simulink model "aIEEE13bus_with_solar_13bus_pl_1day"  (R2025a)
settings: Solver=ode4  StartTime=0.0  StopTime=168  FixedStep=5e-6  MaxStep=1e-4  RelTol=1e-4
InitFcn:
  | a=1; % Loading Factor
  | Ts=50e-6;
  | % phase to sequence conversion of RXB matrices
  | c=1*exp(sqrt(-1)*(120*pi/180));
  | T=[1 1 1;1 c*c c;1 c c*c];
  | Tinv=1/3*[1 1 1;1 c c*c;1 c*c c];
  | 
  | % Simulation data for the IEEE 13 Node Test Feeder model
  | mi2km = 1.60934;%  miles to km conversion
  | ft2km = 0.0003048; % feet to km conversion
  | ms2F = 1*1e-6/(2*pi*60);% microsiemens to Farads conversion
  | 
  | 
  | %% Configuration 601
  | % Series Resitance and Reactance - ohm/mile
  | R_601 = [0.3465 0.1560 0.1580;0.1560 0.3375 0.1535;0.1580 0.1535 0.3414];
  | X_601 = [1.1079 0.5017 0.4236;0.5017 1.0478 0.3849;0.4236 0.3849 1.0348];
  | % charging susceptance - microsiemens/mile
  | B_601 = [6.2998 -1.9958 -1.2595;-1.9958 5.9597 -0.7417;-1.2595 -0.7417 5.6386];
  | 
  | R_601 = R_601/mi2km;
  | Rseq=Tinv*R_601*T;
  | R1_601=Rseq(2,2);R0_601=Rseq(1,1);
  | 
  | L_601 = (X_601/(2*pi*60))/mi2km;
  | Lseq=Tinv*L_601*T;
  | L1_601=Lseq(2,2);L0_601=Lseq(1,1);
  | 
  | C_601 =(B_601*ms2F)/mi2km;
  | Cseq=Tinv*C_601*T;
  | C1_601=Cseq(2,2);C0_601=Cseq(1,1);
  | 
  | %% Configuration 602 - series reactance - ohm/mile
  | R_602 = [0.7526 0.1580 0.1560;0.1580 0.7475 0.1535;0.1560 0.1535 0.7436];
  | X_602 = [1.1814 0.4236 0.5017;0.4236 1.1983 0.3849;0.5017 0.3849 1.2112];
  | % charging susceptance - microsiemens/mile
  | B_602 = [5.6990 -1.0817 -1.6905;-1.0817 5.1795 -0.6588;-1.6905 -0.6588 5.4246];
  | 
  | R_602 = R_602/mi2km;
  | Rseq=Tinv*R_602*T;
  | R1_602=Rseq(2,2);R0_602=Rseq(1,1);
  | 
  | L_602 = (X_602/(2*pi*60))/mi2km;
  | Lseq=Tinv*L_602*T;
  | L1_602=Lseq(2,2);L0_602=Lseq(1,1);
  | 
  | C_602 =(B_602*ms2F)/mi2km;
  | Cseq=Tinv*C_602*T;
  | C1_602=Cseq(2,2);C0_602=Cseq(1,1);
  | %% Configuration 603 - series reactance - ohm/mile
  | R_603 = [0 0 0;0 1.3294 0.2066;0 0.2066 1.3238];
  | X_603 = [0 0 0;0 1.3471 0.4591;0 0.4591 1.3569];
  | % charging susceptance - microsiemens/mile
  | B_603 = [0 0 0;0 4.7097 -0.8999;0 -0.8999 4.6658];
  | 
  | % convert for SPS
  | R_603 = R_603/mi2km;
  | Rseq=Tinv*R_603*T;
  | R1_603=Rseq(2,2);R0_603=Rseq(1,1);
  | 
  | ... (+71 lines)
undefined symbols (not defined in the file or in its folder): D1, Delta, find_system, gcbh, sps_rtmsupport, Ts_Control, Ts_Power
libraries: spsSeriesRLCBranchLib x93, spsGroundLib x57, spsVoltageMeasurementLib x52, spsFourierLib x30, spsThreePhaseVIMeasurementLib x28, spsControlledCurrentSourceLib x25, spsVIMeasurementModel x21, slpidlib x16, spsabctodq0Lib x16, spsCurrentMeasurementLib x11, spsPower3phPhasorLib x11, spsThreePhaseSeriesRLCLoadLib x9
(part 5 of 9)

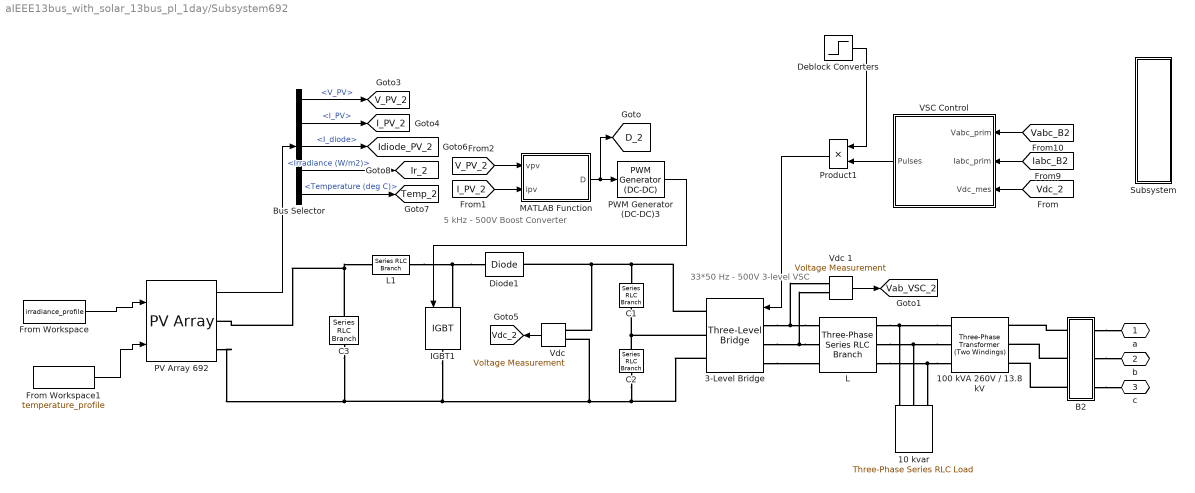
== system aIEEE13bus_with_solar_13bus_pl_1day/Subsystem692 ==
  note: 5 kHz - 500V
      | Boost Converter
  note: 33*50 Hz - 500V
      | 3-level VSC
  10 kvar : spsThreePhaseSeriesRLCLoadLib/Three-Phase Series RLC Load  LConnTagsString=A|B|C  Configuration=Y (grounded)  NominalVoltage=240  Vabc=[1e3 1e3 1e3]  Vabcp=[1e3 1e3 1e3]  NominalFrequency=50  UnbalancedPower=off  ActivePower=10e3/100  InductivePower=0  CapacitivePower=10e3  Pabc=[10e3 9e3 11e3]  QLabc=[100 90 110]  QCabc=[100 90 110]  Pabcp=[10e3 9e3 11e3]  QLabcp=[100 90 110]  QCabcp=[100 90 110]  Measurements=None  LoadType=constant Z
  100 kVA 260V / 13.8 kV : spsThreePhaseTransformerTwoWindingsLib/Three-Phase Transformer (Two Windings)  Winding1Connection=Yg  Winding2Connection=Delta (D1)  CoreType=Three single-phase transformers  SetSaturation=off  Hysteresis=off  DataFile='hysteresis'  SetInitialFlux=off  Measurements=None  UNITS=pu  NominalPower=[100e3 , 50 ]  Winding1=[ 13.8e3 , 0.001 , 0.03 ]  Winding2=[ 260 , 0.001 , 0.03 ]  Rm=500  Lm=500  L0=0.5  Saturation=[ 0,0 ; 0.0024,1.2 ; 1.0,1.52 ]  InitialFluxes=[ 0.8 , -0.8 , 0.7 ]  BreakLoop=off  DiscreteSolver=Trapezoidal iterative  DataType=off  TransfoNumber=0
  3-Level Bridge : spsThreeLevelBridgeLib/Three-Level Bridge  Arms=3  SnubberResistance=1e6  SbubberCapacitance=inf  Device=IGBT / Diodes  Ron=0.2e-3  ForwardVoltages="[  0  0 ]"  Measurements=None
      settings: AttributesFormatString=\n
  B2 : Subsystem  LoadFcn=|  StartFcn=sps_rtmsupport('StartFcn',gcbh);  StopFcn=sps_rtmsupport('StopFcn',gcbh);  mask(Three-Phase VI Measurement){VoltageMeasurement=phase-to-ground, SetLabelV=on, LabelV=Vabc_B2, Vpu=off, VpuLL=off, CurrentMeasurement=yes, SetLabelI=on, LabelI=Iabc_B2, Ipu=off, Pbase=100e6, Vbase=500e3, OutputType=Magnitude, PhasorSimulation=off, PSBequivalent=0}
      | if ~strcmp(get_param(bdroot,'BlockDiagramType'),'library')
      |     set_param([gcb,'/Model'],'LinkStatus','restore');
      | end
      | sps_rtmsupport('LoadFcn',gcbh);
      mask prompts: VoltageMeasurement "Voltage measurement"; SetLabelV "Use a label"; LabelV "Signal label  (use a From block to collect this signal)"; Vpu "Voltages in pu,  based on peak value of nominal phase-to-ground voltage"; VpuLL "Voltages in pu,  based on peak value of nominal phase-to-phase  voltage"; CurrentMeasurement "Current measurement"; SetLabelI "Use a label"; LabelI "Signal label  (use a From block to collect this signal)"; Ipu "Currents in pu"; Pbase "Base power ( VA 3 phase)"; Vbase "Nominal voltage used for pu measurement (Vrms phase-phase) :"; OutputType "Output signals in:"; PhasorSimulation "Phasor simulation (internal use)"; PSBequivalent "Equivalent circuit (internal use)"
      mask help:
      | Ideal three-phase voltage and current measurements.
      |
      | The block can output the voltages and currents in per unit values or in volts and amperes.
      mask init: same as aIEEE13bus_with_solar_13bus_pl_1day/Subsystem611/B3
      settings: CopyFcn=sps_rtmsupport('CopyFcn',gcbh); powericon('ThreePhaseVIMeasurementCopy',gcb)  DeleteFcn=sps_rtmsupport('DeleteFcn',gcbh);  UndoDeleteFcn=sps_rtmsupport('UndoDeleteFcn',gcbh);  ModelCloseFcn=sps_rtmsupport('ModelCloseFcn',gcbh);  PostSaveFcn=sps_rtmsupport('PostSaveFcn',gcbh);  NameChangeFcn=sps_rtmsupport('NameChangeFcn',gcbh);  PreCopyFcn=sps_rtmsupport('PreCopyFcn',gcbh);  OpenFcn=sps_rtmsupport('OpenFcn',gcbh, [1 2 4 5 6 7 9 -12 13]);  CloseFcn=sps_rtmsupport('CloseFcn',gcbh);  PreDeleteFcn=sps_rtmsupport('PreDeleteFcn',gcbh);
      settings: PreSaveFcn=|
      | sps_rtmsupport('PreSaveFcn',gcbh);
      | if ~strcmp(get_param(bdroot(gcbh),'BlockDiagramType'),'library')
      |     set_param(gcb,'LinkStatus','restore')
      | end
      mask Help: helpview(psbhelp)
      mask TypeOptions VoltageMeasurement: no | phase-to-ground | phase-to-phase
      mask Callback VoltageMeasurement: powericon('ThreePhaseVIMeasurementCback',gcb,'Vselector');
      mask Callback SetLabelV: powericon('ThreePhaseVIMeasurementCback',gcb,'');
      mask Callback Vpu: powericon('ThreePhaseVIMeasurementCback',gcb,'Vpu');
      mask Callback VpuLL: powericon('ThreePhaseVIMeasurementCback',gcb,'VpuLL');
      mask TypeOptions CurrentMeasurement: no | yes
      mask Callback CurrentMeasurement: powericon('ThreePhaseVIMeasurementCback',gcb,'');
      mask Callback SetLabelI: powericon('ThreePhaseVIMeasurementCback',gcb,'');
      mask Callback LabelI: powericon('ThreePhaseVIMeasurementCback',gcb,'');
      mask Callback Ipu: powericon('ThreePhaseVIMeasurementCback',gcb,'');
      mask TypeOptions OutputType: Complex | Real-Imag | Magnitude-Angle | Magnitude
  Bus Selector : BusSelector  OutputSignals=V_PV,I_PV,I_diode,Irradiance (W/m2),Temperature (deg C)
  C1 : spsSeriesRLCBranchLib/Series RLC Branch  LConnTagsString=__new0  RConnTagsString=__new0  BranchType=C  Resistance=1.0  Inductance=1.0  SetiL0=off  InitialCurrent=0  Capacitance=12000e-06  Setx0=off  InitialVoltage=0  Measurements=None
  C2 : spsSeriesRLCBranchLib/Series RLC Branch  LConnTagsString=__new0  RConnTagsString=__new0  BranchType=C  Resistance=1.0  Inductance=1.0  SetiL0=off  InitialCurrent=0  Capacitance=12000e-06  Setx0=off  InitialVoltage=0  Measurements=None
  C3 : spsSeriesRLCBranchLib/Series RLC Branch  LConnTagsString=__new0  RConnTagsString=__new0  BranchType=C  Resistance=1.0  Inductance=1.0  SetiL0=off  InitialCurrent=0  Capacitance=100e-6  Setx0=off  InitialVoltage=0  Measurements=Branch voltage
  Deblock Converters : Step  Time=0.05  SampleTime=0
  Diode1 : spsDiodeLib/Diode  Ron=1e-4  Lon=0  Vf=0  IC=0  UseSnubber=off  Rs=inf  Cs=inf  Measurements=off
  From Workspace : FromWorkspace  VariableName=irradiance_profile  SampleTime=-1  OutputAfterFinalValue=Holding final value
  From Workspace1 : FromWorkspace  VariableName=temperature_profile  SampleTime=-1  OutputAfterFinalValue=Holding final value
  IGBT1 : spsIGBTLib/IGBT  Ron=0.001  Lon=0  Vf=0  Tf=0  Tt=0  IC=0  Rs=1e5  Cs=inf  Measurements=off
  L : spsThreePhaseSeriesRLCBranchLib/Three-Phase Series RLC Branch  LConnTagsString=A|B|C  RConnTagsString=A|B|C  BranchType=RL  Resistance=500e-6*377/50/2  Inductance=500e-6/2  Capacitance=inf  Measurements=None
  L1 : spsSeriesRLCBranchLib/Series RLC Branch  LConnTagsString=__new0  RConnTagsString=__new0  BranchType=RL  Resistance=0.005  Inductance=5e-3  SetiL0=off  InitialCurrent=0  Capacitance=1e-6  Setx0=off  InitialVoltage=0  Measurements=None
  MATLAB Function : MATLAB Function  TreatAsAtomicUnit=on
  PV Array 692 : spsPVArrayLib/PV Array  Npar=8  Nser=23  PlotType=array @ 1000 W/m2 & specified temperatures  S_vec="[ 1000  500  100 ]"  Temp_C_vec="[ 45 25  ]"  ModuleName=User-defined  PlotWhenSelected=off  Pm=550.44  Ncell=60  Voc=49.5  Isc=14  Vm=41.7  Im=13.2  beta_Voc_pc=-0.143  alpha_Isc_pc=0.007  beta_Voc=-0.070785  alpha_Isc=0.00098  IL=14.1256  I0=7.3977e-15  nI=0.91366  Rsh=88.9397  Rs=0.23098  RobustModel=off  RobustCellTemperature=313.3991  BAL=on  Tc=1e-6  Tfilter=5e-5
  PWM Generator (DC-DC)3 : spsPWMGeneratorDCDCLib/PWM Generator (DC-DC)  Fsw=5000  Ts=5e-6
  Product1 : Product  RndMeth=Zero
  Subsystem : Subsystem
  VSC Control : Subsystem  mask(VSC Main Controller){nom=[ 100e3  50 ], Vnom=[ 25e3 260 ], Vnom_dc=500, RLxfo=[0.002  0.06 ], RLchoke=[2e-3  250e-6  ], K_VDCreg=[7  800], K_Ireg=[0.3 20], Ts=0.001}
      mask prompts: nom "Nominal power and frequency [ Pnom(VA)  Fnom(Hz) ]:"; Vnom "Nominal primary and secondary voltages (Vrms LL) [ Vnom_prim   Vnom_sec ]:"; Vnom_dc "Nominal DC bus voltage (V):"; RLxfo "Total transformer leakage impedance (pu/Pnom) [ Rxfo  Lxf ]"; RLchoke "Choke impedance [ R(ohm) L(H) ]"; K_VDCreg "VDC regultator gains [ Kp  Ki ]:"; K_Ireg "Current regulator gains [ Kp  Ki ]:"; Ts "Sample time"
      mask init: same as aIEEE13bus_with_solar_13bus_pl_1day/Subsystem611/VSC Control
  "Vdc " : spsVoltageMeasurementLib/Voltage Measurement  Tag=PoWeRsYsTeMmEaSuReMeNt  PhasorSimulation=off  OutputType=Magnitude  PSBequivalent=0
  Vdc 1 : spsVoltageMeasurementLib/Voltage Measurement  Tag=PoWeRsYsTeMmEaSuReMeNt  PhasorSimulation=off  OutputType=Magnitude  PSBequivalent=0
  a : PMIOPort  Side=Right
  b : PMIOPort  Port=2  Side=Right
  c : PMIOPort  Port=3  Side=Right
  tag scope: D_2=global, I_PV_2=global, Idiode_PV_2=global, Ir_2=global, Temp_2=global, V_PV_2=global, Vab_VSC_2=global, Vdc_2=global
  wires:
  [Vdc_2] -> VSC Control/3(Vdc_mes)
  From Workspace1/1 -> PV Array 692/2
  MATLAB Function/1(D) -> [D_2], PWM Generator (DC-DC)3/1
  Bus Selector/3 -> [Idiode_PV_2]  "<I_diode>"
  Bus Selector/4 -> [Ir_2]  "<Irradiance (W/m2)>"
  [Vabc_B2] -> VSC Control/1(Vabc_prim)
  Bus Selector/2 -> [I_PV_2]  "<I_PV>"
  Bus Selector/5 -> [Temp_2]  "<Temperature (deg C)>"
  Deblock Converters/1 -> Product1/1
  Product1/1 -> 3-Level Bridge/1
  Bus Selector/1 -> [V_PV_2]  "<V_PV>"
  Vdc 1/1 -> [Vab_VSC_2]
  [Iabc_B2] -> VSC Control/2(Iabc_prim)
  [I_PV_2] -> MATLAB Function/2(ipv)
  From Workspace/1 -> PV Array 692/1
  PV Array 692/1 -> Bus Selector/1
  "Vdc "/1 -> [Vdc_2]
  VSC Control/1(Pulses) -> Product1/2
  [V_PV_2] -> MATLAB Function/1(vpv)
  PWM Generator (DC-DC)3/1 -> IGBT1/1
  connections:
  B2/RConn3 -- c/RConn1
  Diode1/LConn1 -- IGBT1/LConn1 -- L1/RConn1
  100 kVA 260V / 13.8 kV/RConn1 -- 10 kvar/LConn1 -- L/RConn1
  L/LConn2 -- Vdc 1/LConn2 -- 3-Level Bridge/LConn2
  3-Level Bridge/LConn3 -- L/LConn3
  IGBT1/RConn1 -- 3-Level Bridge/RConn3 -- C2/RConn1 -- "Vdc "/LConn2 -- PV Array 692/RConn2 -- C3/RConn1
  B2/LConn1 -- 100 kVA 260V / 13.8 kV/LConn1
  100 kVA 260V / 13.8 kV/RConn2 -- 10 kvar/LConn2 -- L/RConn2
  100 kVA 260V / 13.8 kV/RConn3 -- 10 kvar/LConn3 -- L/RConn3
  C3/LConn1 -- PV Array 692/RConn1 -- L1/LConn1
  B2/LConn2 -- 100 kVA 260V / 13.8 kV/LConn2
  C1/RConn1 -- 3-Level Bridge/RConn2 -- C2/LConn1
  L/LConn1 -- Vdc 1/LConn1 -- 3-Level Bridge/LConn1
  B2/LConn3 -- 100 kVA 260V / 13.8 kV/LConn3
  "Vdc "/LConn1 -- C1/LConn1 -- 3-Level Bridge/RConn1 -- Diode1/RConn1
  B2/RConn1 -- a/RConn1
  B2/RConn2 -- b/RConn1

== system aIEEE13bus_with_solar_13bus_pl_1day/Regulator 1/Single Phase SVR_A ==
  Line Drop Compensator : Subsystem
  Transformer with Taps : Subsystem
  Voltage Regulator Control : Subsystem
  S : PMIOPort  Tag=PMCPort  Side=Left
  L : PMIOPort  Tag=PMCPort  Port=2  Side=Right
  Tap : Outport  VectorParamsAs1DForOutWhenUnconnected=off
  tag scope: Vr1a=global
  wires:
  Line Drop Compensator/1(Vm) -> Voltage Regulator Control/1(Vm), [Vr1a]
  Voltage Regulator Control/2(Tap) -> Tap/1
  Voltage Regulator Control/1(N) -> Transformer with Taps/1(N)
  Transformer with Taps/1(Isec) -> Line Drop Compensator/1(Isec)
  Transformer with Taps/2(Vsec) -> Line Drop Compensator/2(Vsec)
  connections:
  Transformer with Taps/RConn1 -- L/RConn1
  S/RConn1 -- Transformer with Taps/LConn1

== system aIEEE13bus_with_solar_13bus_pl_1day/Regulator 1/Single Phase SVR_B ==
  Line Drop Compensator : Subsystem
  Transformer with Taps : Subsystem
  Voltage Regulator Control : Subsystem
  S : PMIOPort  Tag=PMCPort  Side=Left
  L : PMIOPort  Tag=PMCPort  Port=2  Side=Right
  Tap : Outport  VectorParamsAs1DForOutWhenUnconnected=off
  tag scope: Vr1b=global
  wires:
  Transformer with Taps/2(Vsec) -> Line Drop Compensator/2(Vsec)
  Transformer with Taps/1(Isec) -> Line Drop Compensator/1(Isec)
  Voltage Regulator Control/1(N) -> Transformer with Taps/1(N)
  Voltage Regulator Control/2(Tap) -> Tap/1
  Line Drop Compensator/1(Vm) -> [Vr1b], Voltage Regulator Control/1(Vm)
  connections:
  S/RConn1 -- Transformer with Taps/LConn1
  Transformer with Taps/RConn1 -- L/RConn1

== system aIEEE13bus_with_solar_13bus_pl_1day/Regulator 1/Single Phase SVR_C ==
  Line Drop Compensator : Subsystem
  Transformer with Taps : Subsystem
  Voltage Regulator Control : Subsystem
  S : PMIOPort  Tag=PMCPort  Side=Left
  L : PMIOPort  Tag=PMCPort  Port=2  Side=Right
  Tap : Outport  VectorParamsAs1DForOutWhenUnconnected=off
  tag scope: Vr1c=global
  wires:
  Line Drop Compensator/1(Vm) -> Voltage Regulator Control/1(Vm), [Vr1c]
  Voltage Regulator Control/2(Tap) -> Tap/1
  Voltage Regulator Control/1(N) -> Transformer with Taps/1(N)
  Transformer with Taps/1(Isec) -> Line Drop Compensator/1(Isec)
  Transformer with Taps/2(Vsec) -> Line Drop Compensator/2(Vsec)
  connections:
  Transformer with Taps/RConn1 -- L/RConn1
  S/RConn1 -- Transformer with Taps/LConn1

== system aIEEE13bus_with_solar_13bus_pl_1day/Subsystem611/B3 ==
  Kv : Gain  Gain=Ki  SaturateOnIntegerOverflow=on  OutDataTypeStr=Inherit: Same as input  ParamDataTypeStr=Inherit: Same as input
  Kv1 : Gain  Gain=Kv  SaturateOnIntegerOverflow=on  OutDataTypeStr=Inherit: Same as input  ParamDataTypeStr=Inherit: Same as input
  Mode I : spsVIMeasurementModel/Complex  SystemSampleTime=-1  VariantActivationTime=update diagram  EmptyChoice=off  PassThrough=off  PassThroughVariantControl=(default)  EmptyChoiceVariantControl=(default)  AllowFlexibleInterface=on  Latency=0  AutoFrameSizeCalculation=off
  Mode V : spsVIMeasurementModel/Complex  SystemSampleTime=-1  VariantActivationTime=update diagram  EmptyChoice=off  PassThrough=off  PassThroughVariantControl=(default)  EmptyChoiceVariantControl=(default)  AllowFlexibleInterface=on  Latency=0  AutoFrameSizeCalculation=off
  Model : spsVIMeasurementModel/VI  SystemSampleTime=-1  VariantActivationTime=update diagram  EmptyChoice=off  PassThrough=off  PassThroughVariantControl=(default)  EmptyChoiceVariantControl=(default)  AllowFlexibleInterface=on  Latency=0  AutoFrameSizeCalculation=off
  A : PMIOPort  Side=Left
  B : PMIOPort  Port=2  Side=Left
  C : PMIOPort  Port=3  Side=Left
  a : PMIOPort  Port=4  Side=Right
  b : PMIOPort  Port=5  Side=Right
  c : PMIOPort  Port=6  Side=Right
  tag scope: Iabc_B3=global, Vabc_B3=global
  wires:
  Mode V/1 -> [Vabc_B3]
  Mode I/1 -> [Iabc_B3]
  Kv1/1 -> Mode V/1
  Kv/1 -> Mode I/1
  Model/1 -> Kv1/1
  Model/2 -> Kv/1
  connections:
  Model/LConn2 -- B/RConn1
  Model/LConn1 -- A/RConn1
  Model/LConn3 -- C/RConn1
  Model/RConn2 -- b/RConn1
  Model/RConn1 -- a/RConn1
  Model/RConn3 -- c/RConn1

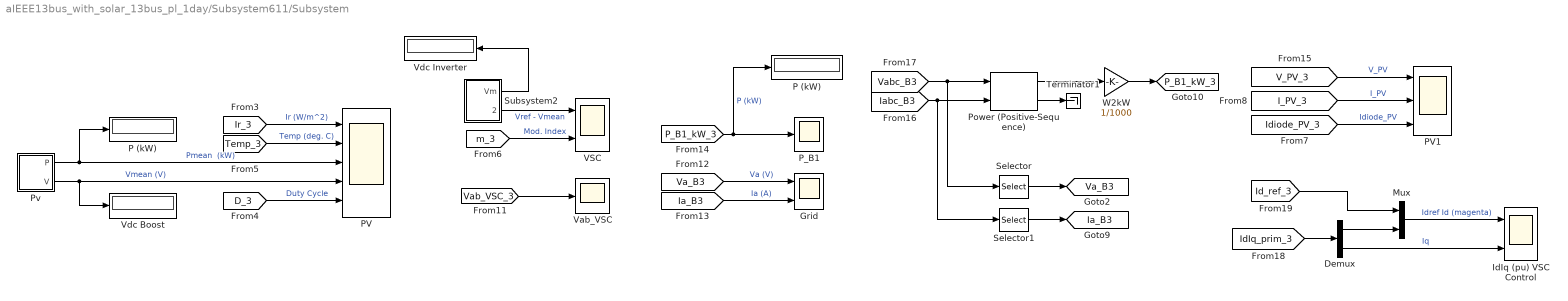
== system aIEEE13bus_with_solar_13bus_pl_1day/Subsystem611/Subsystem ==
  Demux : Demux  Outputs=2
  Grid : Scope  NumInputPorts=2
      settings: TimeSpan=0.05  ActiveDisplayYMinimum=-15250.872  ActiveDisplayYMaximum=15249.0697  DataLoggingDecimation=20  DataLoggingSaveFormat=Array
  IdIq (pu) VSC Control : Scope  NumInputPorts=2
      settings: TimeSpan=2  ActiveDisplayYMinimum=-5  ActiveDisplayYMaximum=5  DataLoggingDecimation=100  DataLoggingVariableName=ScopeData2  DataLoggingSaveFormat=Array
  Mux : Mux  Inputs=2
  P (kW) : Display
      settings: Format=bank  Decimation=2000
  "P (kW) " : Display
      settings: Format=bank  Decimation=2000
  PV : Scope  NumInputPorts=5
      settings: TimeSpan=2.5  ActiveDisplayYMinimum=156.25  ActiveDisplayYMaximum=1093.75  DataLoggingDecimation=100  DataLoggingVariableName=ScopeData3  DataLoggingSaveFormat=Array
  PV1 : Scope  NumInputPorts=3
      settings: TimeSpan=2  ActiveDisplayYMinimum=-37.8929  ActiveDisplayYMaximum=360.8644  DataLoggingDecimation=100  DataLoggingVariableName=ScopeData4  DataLoggingSaveFormat=Array
  P_B1 : Scope
      settings: TimeSpan=2.5  ActiveDisplayYMinimum=-54.8007  ActiveDisplayYMaximum=191.472  DataLoggingDecimation=100  DataLoggingVariableName=ScopeData5  DataLoggingSaveFormat=Array
  Power (Positive-Sequence) : spsPowerPositiveSequenceLib/Power (Positive-Sequence)  Freq=60  Vinit=[0, 0]  Iinit=[0, 0]  Ts=Ts_Control
  Pv : Subsystem
  Selector : Selector  InputPortWidth=3  IndexOptions=Index vector (dialog)  Indices=[1]  OutputSizes=1
  Selector1 : Selector  InputPortWidth=3  IndexOptions=Index vector (dialog)  Indices=[1]  OutputSizes=1
  Subsystem2 : Subsystem
  Terminator1 : Terminator
  VSC : Scope  NumInputPorts=2
      settings: TimeSpan=2.5  ActiveDisplayYMinimum=-145.1969  ActiveDisplayYMaximum=1306.7724  DataLoggingDecimation=100  DataLoggingVariableName=ScopeData6  DataLoggingSaveFormat=Array
  Vab_VSC : Scope
      settings: ActiveDisplayYMinimum=-833.7525  ActiveDisplayYMaximum=1202.9579  DataLoggingDecimation=10  DataLoggingVariableName=ScopeData7  DataLoggingSaveFormat=Array
  Vdc Boost : Display
      settings: Format=bank  Decimation=2000
  Vdc Inverter : Display
      settings: Format=bank  Decimation=2000
  W2kW : Gain  Gain=1/1000
  tag scope: Ia_B3=global, P_B1_kW_3=global, Va_B3=global
  wires:
  Selector/1 -> [Va_B3]
  [IdIq_prim_3] -> Demux/1
  [D_3] -> PV/5  "Duty Cycle"
  Pv/2(V) -> Vdc Boost/1, PV/4  "Vmean (V)"
  Selector1/1 -> [Ia_B3]
  [Temp_3] -> PV/2  "Temp (deg. C)"
  [Id_ref_3] -> Mux/1
  Power (Positive-Sequence)/2 -> Terminator1/1
  Pv/1(P) -> "P (kW) "/1, PV/3  "Pmean  (kW)"
  Power (Positive-Sequence)/1 -> W2kW/1
  [Va_B3] -> Grid/1  "Va (V)"
  [P_B1_kW_3] -> P_B1/1, P (kW)/1  "P (kW)"
  [Iabc_B3] -> Power (Positive-Sequence)/2, Selector1/1
  [Vab_VSC_3] -> Vab_VSC/1
  Demux/2 -> IdIq (pu) VSC Control/2  "Iq"
  Subsystem2/2(VrVm) -> VSC/1  "Vref - Vmean"
  [Vabc_B3] -> Power (Positive-Sequence)/1, Selector/1
  [m_3] -> VSC/2  "Mod. Index"
  Subsystem2/1(Vm) -> Vdc Inverter/1
  [V_PV_3] -> PV1/1  "V_PV"
  [I_PV_3] -> PV1/2  "I_PV"
  Mux/1 -> IdIq (pu) VSC Control/1  "Idref Id (magenta)"
  [Ia_B3] -> Grid/2  "Ia (A)"
  Demux/1 -> Mux/2
  W2kW/1 -> [P_B1_kW_3]
  [Ir_3] -> PV/1  "Ir (W/m^2)"
  [Idiode_PV_3] -> PV1/3  "Idiode_PV"

== system aIEEE13bus_with_solar_13bus_pl_1day/Subsystem611/VSC Control ==
  note: VSC Main Controller
  Vabc_prim : Inport  PortDimensions=3
  Iabc_prim : Inport  Port=2  PortDimensions=3
  Vdc_mes : Inport  Port=3  PortDimensions=1
  Current Regulator : Subsystem
  Iq_ref : Constant  Value=0
  Mux : Mux  Inputs=2
  PLL & Measurements : Subsystem
  PWM Generator (3-Level) : spsPWMGenerator3LevelLib/PWM Generator (3-Level)  ModulatorType=Three-phase bridge (12 pulses)  ModulatorMode=Unsynchronized  nF=27  Fc=33*60  ModulatingSignals=off  m=0.8  Freq=60  Phase=0  Ts=Ts_Power
  Uabc_ref Generation max (m) = 1 : Subsystem
  Unit Delay : UnitDelay  SampleTime=Ts_Control  HasFrameUpgradeWarning=on
  VDC Regulator : Subsystem
  Vdc_ref1 : Constant  Value=Vdc_ref
  Pulses : Outport  VectorParamsAs1DForOutWhenUnconnected=off
  wires:
  VDC Regulator/1(Id_ref) -> Mux/1
  PLL & Measurements/1(wt) -> Uabc_ref Generation max (m) = 1/1(wt)
  Current Regulator/1(VdVq_conv) -> Uabc_ref Generation max (m) = 1/2(VdVq_conv)
  Iq_ref/1 -> Mux/2
  Mux/1 -> Current Regulator/3(IdIq_ref)
  PLL & Measurements/3(IdIq_prim) -> Current Regulator/2(IdIq_mes)
  PLL & Measurements/2(VdVq_prim) -> Current Regulator/1(VdVq_mes)
  Vdc_mes/1 -> VDC Regulator/1(Vdc_mes)
  Vabc_prim/1 -> PLL & Measurements/1(Vabc_prim)
  Iabc_prim/1 -> PLL & Measurements/2(Iabc_prim)
  Unit Delay/1 -> PWM Generator (3-Level)/1
  PWM Generator (3-Level)/1 -> Pulses/1
  Uabc_ref Generation max (m) = 1/1(Uabc_ref) -> Unit Delay/1
  Vdc_ref1/1 -> VDC Regulator/2(Vdc_ref)

== system aIEEE13bus_with_solar_13bus_pl_1day/Subsystem634/B4 ==
  Kv : Gain  Gain=Ki  SaturateOnIntegerOverflow=on  OutDataTypeStr=Inherit: Same as input  ParamDataTypeStr=Inherit: Same as input
  Kv1 : Gain  Gain=Kv  SaturateOnIntegerOverflow=on  OutDataTypeStr=Inherit: Same as input  ParamDataTypeStr=Inherit: Same as input
  Mode I : spsVIMeasurementModel/Complex  SystemSampleTime=-1  VariantActivationTime=update diagram  EmptyChoice=off  PassThrough=off  PassThroughVariantControl=(default)  EmptyChoiceVariantControl=(default)  AllowFlexibleInterface=on  Latency=0  AutoFrameSizeCalculation=off
  Mode V : spsVIMeasurementModel/Complex  SystemSampleTime=-1  VariantActivationTime=update diagram  EmptyChoice=off  PassThrough=off  PassThroughVariantControl=(default)  EmptyChoiceVariantControl=(default)  AllowFlexibleInterface=on  Latency=0  AutoFrameSizeCalculation=off
  Model : spsVIMeasurementModel/VI  SystemSampleTime=-1  VariantActivationTime=update diagram  EmptyChoice=off  PassThrough=off  PassThroughVariantControl=(default)  EmptyChoiceVariantControl=(default)  AllowFlexibleInterface=on  Latency=0  AutoFrameSizeCalculation=off
  A : PMIOPort  Side=Left
  B : PMIOPort  Port=2  Side=Left
  C : PMIOPort  Port=3  Side=Left
  a : PMIOPort  Port=4  Side=Right
  b : PMIOPort  Port=5  Side=Right
  c : PMIOPort  Port=6  Side=Right
  tag scope: Iabc_B4=global, Vabc_B4=global
  wires:
  Mode V/1 -> [Vabc_B4]
  Mode I/1 -> [Iabc_B4]
  Kv1/1 -> Mode V/1
  Kv/1 -> Mode I/1
  Model/1 -> Kv1/1
  Model/2 -> Kv/1
  connections:
  Model/LConn2 -- B/RConn1
  Model/LConn1 -- A/RConn1
  Model/LConn3 -- C/RConn1
  Model/RConn2 -- b/RConn1
  Model/RConn1 -- a/RConn1
  Model/RConn3 -- c/RConn1

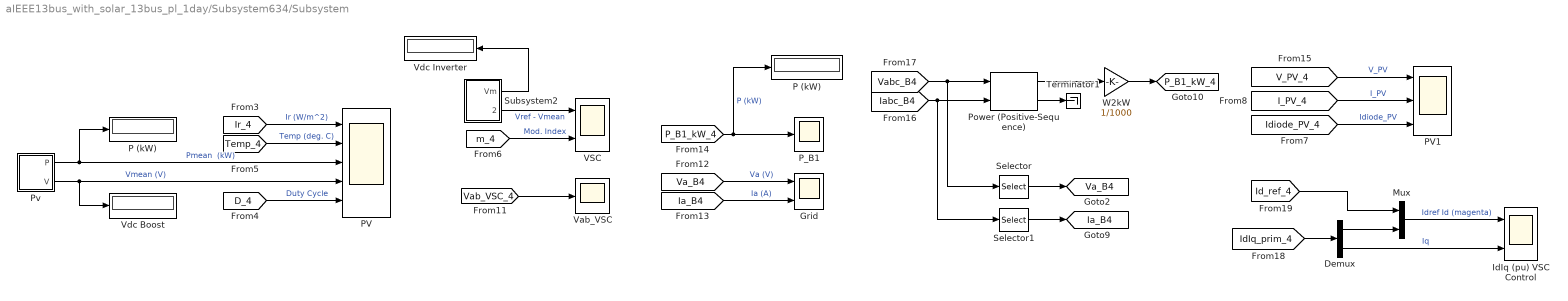
== system aIEEE13bus_with_solar_13bus_pl_1day/Subsystem634/Subsystem ==
  Demux : Demux  Outputs=2
  Grid : Scope  NumInputPorts=2
      settings: TimeSpan=0.05  ActiveDisplayYMinimum=-15250.872  ActiveDisplayYMaximum=15249.0697  DataLoggingDecimation=20  DataLoggingSaveFormat=Array
  IdIq (pu) VSC Control : Scope  NumInputPorts=2
      settings: TimeSpan=2  ActiveDisplayYMinimum=-5  ActiveDisplayYMaximum=5  DataLoggingDecimation=100  DataLoggingVariableName=ScopeData2  DataLoggingSaveFormat=Array
  Mux : Mux  Inputs=2
  P (kW) : Display
      settings: Format=bank  Decimation=2000
  "P (kW) " : Display
      settings: Format=bank  Decimation=2000
  PV : Scope  NumInputPorts=5
      settings: TimeSpan=2.5  ActiveDisplayYMinimum=156.25  ActiveDisplayYMaximum=1093.75  DataLoggingDecimation=100  DataLoggingVariableName=ScopeData3  DataLoggingSaveFormat=Array
  PV1 : Scope  NumInputPorts=3
      settings: TimeSpan=2  ActiveDisplayYMinimum=-37.8929  ActiveDisplayYMaximum=360.8644  DataLoggingDecimation=100  DataLoggingVariableName=ScopeData4  DataLoggingSaveFormat=Array
  P_B1 : Scope
      settings: TimeSpan=2.5  ActiveDisplayYMinimum=-54.8007  ActiveDisplayYMaximum=191.472  DataLoggingDecimation=100  DataLoggingVariableName=ScopeData5  DataLoggingSaveFormat=Array
  Power (Positive-Sequence) : spsPowerPositiveSequenceLib/Power (Positive-Sequence)  Freq=60  Vinit=[0, 0]  Iinit=[0, 0]  Ts=Ts_Control
  Pv : Subsystem
  Selector : Selector  InputPortWidth=3  IndexOptions=Index vector (dialog)  Indices=[1]  OutputSizes=1
  Selector1 : Selector  InputPortWidth=3  IndexOptions=Index vector (dialog)  Indices=[1]  OutputSizes=1
  Subsystem2 : Subsystem
  Terminator1 : Terminator
  VSC : Scope  NumInputPorts=2
      settings: TimeSpan=2.5  ActiveDisplayYMinimum=-145.1969  ActiveDisplayYMaximum=1306.7724  DataLoggingDecimation=100  DataLoggingVariableName=ScopeData6  DataLoggingSaveFormat=Array
  Vab_VSC : Scope
      settings: ActiveDisplayYMinimum=-833.7525  ActiveDisplayYMaximum=1202.9579  DataLoggingDecimation=10  DataLoggingVariableName=ScopeData7  DataLoggingSaveFormat=Array
  Vdc Boost : Display
      settings: Format=bank  Decimation=2000
  Vdc Inverter : Display
      settings: Format=bank  Decimation=2000
  W2kW : Gain  Gain=1/1000
  tag scope: Ia_B4=global, P_B1_kW_4=global, Va_B4=global
  wires:
  Selector/1 -> [Va_B4]
  [IdIq_prim_4] -> Demux/1
  [D_4] -> PV/5  "Duty Cycle"
  Pv/2(V) -> Vdc Boost/1, PV/4  "Vmean (V)"
  Selector1/1 -> [Ia_B4]
  [Temp_4] -> PV/2  "Temp (deg. C)"
  [Id_ref_4] -> Mux/1
  Power (Positive-Sequence)/2 -> Terminator1/1
  Pv/1(P) -> "P (kW) "/1, PV/3  "Pmean  (kW)"
  Power (Positive-Sequence)/1 -> W2kW/1
  [Va_B4] -> Grid/1  "Va (V)"
  [P_B1_kW_4] -> P_B1/1, P (kW)/1  "P (kW)"
  [Iabc_B4] -> Power (Positive-Sequence)/2, Selector1/1
  [Vab_VSC_4] -> Vab_VSC/1
  Demux/2 -> IdIq (pu) VSC Control/2  "Iq"
  Subsystem2/2(VrVm) -> VSC/1  "Vref - Vmean"
  [Vabc_B4] -> Power (Positive-Sequence)/1, Selector/1
  [m_4] -> VSC/2  "Mod. Index"
  Subsystem2/1(Vm) -> Vdc Inverter/1
  [V_PV_4] -> PV1/1  "V_PV"
  [I_PV_4] -> PV1/2  "I_PV"
  Mux/1 -> IdIq (pu) VSC Control/1  "Idref Id (magenta)"
  [Ia_B4] -> Grid/2  "Ia (A)"
  Demux/1 -> Mux/2
  W2kW/1 -> [P_B1_kW_4]
  [Ir_4] -> PV/1  "Ir (W/m^2)"
  [Idiode_PV_4] -> PV1/3  "Idiode_PV"

== system aIEEE13bus_with_solar_13bus_pl_1day/Subsystem634/VSC Control ==
  note: VSC Main Controller
  Vabc_prim : Inport  PortDimensions=3
  Iabc_prim : Inport  Port=2  PortDimensions=3
  Vdc_mes : Inport  Port=3  PortDimensions=1
  Current Regulator : Subsystem
  Iq_ref : Constant  Value=0
  Mux : Mux  Inputs=2
  PLL & Measurements : Subsystem
  PWM Generator (3-Level) : spsPWMGenerator3LevelLib/PWM Generator (3-Level)  ModulatorType=Three-phase bridge (12 pulses)  ModulatorMode=Unsynchronized  nF=27  Fc=33*60  ModulatingSignals=off  m=0.8  Freq=60  Phase=0  Ts=Ts_Power
  Uabc_ref Generation max (m) = 1 : Subsystem
  Unit Delay : UnitDelay  SampleTime=Ts_Control  HasFrameUpgradeWarning=on
  VDC Regulator : Subsystem
  Vdc_ref1 : Constant  Value=Vdc_ref
  Pulses : Outport  VectorParamsAs1DForOutWhenUnconnected=off
  wires:
  VDC Regulator/1(Id_ref) -> Mux/1
  PLL & Measurements/1(wt) -> Uabc_ref Generation max (m) = 1/1(wt)
  Current Regulator/1(VdVq_conv) -> Uabc_ref Generation max (m) = 1/2(VdVq_conv)
  Iq_ref/1 -> Mux/2
  Mux/1 -> Current Regulator/3(IdIq_ref)
  PLL & Measurements/3(IdIq_prim) -> Current Regulator/2(IdIq_mes)
  PLL & Measurements/2(VdVq_prim) -> Current Regulator/1(VdVq_mes)
  Vdc_mes/1 -> VDC Regulator/1(Vdc_mes)
  Vabc_prim/1 -> PLL & Measurements/1(Vabc_prim)
  Iabc_prim/1 -> PLL & Measurements/2(Iabc_prim)
  Unit Delay/1 -> PWM Generator (3-Level)/1
  PWM Generator (3-Level)/1 -> Pulses/1
  Uabc_ref Generation max (m) = 1/1(Uabc_ref) -> Unit Delay/1
  Vdc_ref1/1 -> VDC Regulator/2(Vdc_ref)

== system aIEEE13bus_with_solar_13bus_pl_1day/Subsystem645/B5 ==
  Kv : Gain  Gain=Ki  SaturateOnIntegerOverflow=on  OutDataTypeStr=Inherit: Same as input  ParamDataTypeStr=Inherit: Same as input
  Kv1 : Gain  Gain=Kv  SaturateOnIntegerOverflow=on  OutDataTypeStr=Inherit: Same as input  ParamDataTypeStr=Inherit: Same as input
  Mode I : spsVIMeasurementModel/Complex  SystemSampleTime=-1  VariantActivationTime=update diagram  EmptyChoice=off  PassThrough=off  PassThroughVariantControl=(default)  EmptyChoiceVariantControl=(default)  AllowFlexibleInterface=on  Latency=0  AutoFrameSizeCalculation=off
  Mode V : spsVIMeasurementModel/Complex  SystemSampleTime=-1  VariantActivationTime=update diagram  EmptyChoice=off  PassThrough=off  PassThroughVariantControl=(default)  EmptyChoiceVariantControl=(default)  AllowFlexibleInterface=on  Latency=0  AutoFrameSizeCalculation=off
  Model : spsVIMeasurementModel/VI  SystemSampleTime=-1  VariantActivationTime=update diagram  EmptyChoice=off  PassThrough=off  PassThroughVariantControl=(default)  EmptyChoiceVariantControl=(default)  AllowFlexibleInterface=on  Latency=0  AutoFrameSizeCalculation=off
  A : PMIOPort  Side=Left
  B : PMIOPort  Port=2  Side=Left
  C : PMIOPort  Port=3  Side=Left
  a : PMIOPort  Port=4  Side=Right
  b : PMIOPort  Port=5  Side=Right
  c : PMIOPort  Port=6  Side=Right
  tag scope: Iabc_B5=global, Vabc_B5=global
  wires:
  Mode V/1 -> [Vabc_B5]
  Mode I/1 -> [Iabc_B5]
  Kv1/1 -> Mode V/1
  Kv/1 -> Mode I/1
  Model/1 -> Kv1/1
  Model/2 -> Kv/1
  connections:
  Model/LConn2 -- B/RConn1
  Model/LConn1 -- A/RConn1
  Model/LConn3 -- C/RConn1
  Model/RConn2 -- b/RConn1
  Model/RConn1 -- a/RConn1
  Model/RConn3 -- c/RConn1

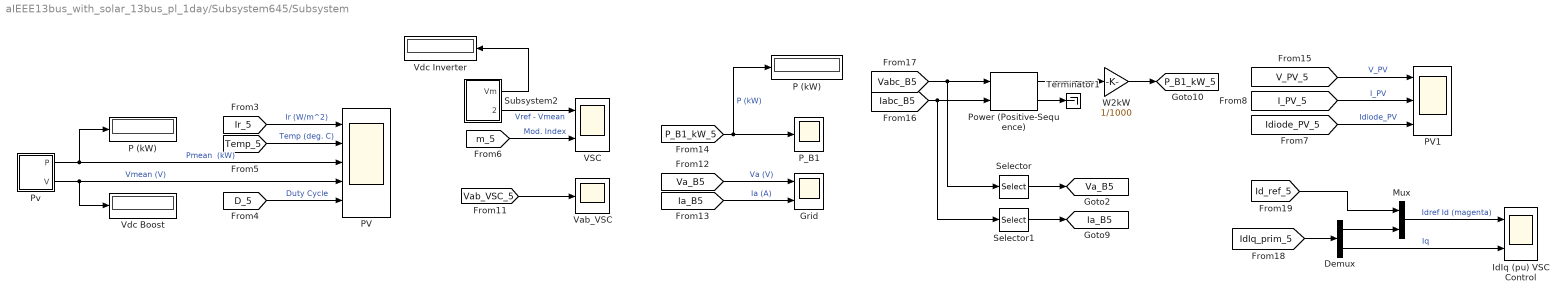
== system aIEEE13bus_with_solar_13bus_pl_1day/Subsystem645/Subsystem ==
  Demux : Demux  Outputs=2
  Grid : Scope  NumInputPorts=2
      settings: TimeSpan=0.05  ActiveDisplayYMinimum=-15250.872  ActiveDisplayYMaximum=15249.0697  DataLoggingDecimation=20  DataLoggingSaveFormat=Array
  IdIq (pu) VSC Control : Scope  NumInputPorts=2
      settings: TimeSpan=2  ActiveDisplayYMinimum=-5  ActiveDisplayYMaximum=5  DataLoggingDecimation=100  DataLoggingVariableName=ScopeData2  DataLoggingSaveFormat=Array
  Mux : Mux  Inputs=2
  P (kW) : Display
      settings: Format=bank  Decimation=2000
  "P (kW) " : Display
      settings: Format=bank  Decimation=2000
  PV : Scope  NumInputPorts=5
      settings: TimeSpan=2.5  ActiveDisplayYMinimum=156.25  ActiveDisplayYMaximum=1093.75  DataLoggingDecimation=100  DataLoggingVariableName=ScopeData3  DataLoggingSaveFormat=Array
  PV1 : Scope  NumInputPorts=3
      settings: TimeSpan=2  ActiveDisplayYMinimum=-37.8929  ActiveDisplayYMaximum=360.8644  DataLoggingDecimation=100  DataLoggingVariableName=ScopeData4  DataLoggingSaveFormat=Array
  P_B1 : Scope
      settings: TimeSpan=2.5  ActiveDisplayYMinimum=-54.8007  ActiveDisplayYMaximum=191.472  DataLoggingDecimation=100  DataLoggingVariableName=ScopeData5  DataLoggingSaveFormat=Array
  Power (Positive-Sequence) : spsPowerPositiveSequenceLib/Power (Positive-Sequence)  Freq=60  Vinit=[0, 0]  Iinit=[0, 0]  Ts=Ts_Control
  Pv : Subsystem
  Selector : Selector  InputPortWidth=3  IndexOptions=Index vector (dialog)  Indices=[1]  OutputSizes=1
  Selector1 : Selector  InputPortWidth=3  IndexOptions=Index vector (dialog)  Indices=[1]  OutputSizes=1
  Subsystem2 : Subsystem
  Terminator1 : Terminator
  VSC : Scope  NumInputPorts=2
      settings: TimeSpan=2.5  ActiveDisplayYMinimum=-145.1969  ActiveDisplayYMaximum=1306.7724  DataLoggingDecimation=100  DataLoggingVariableName=ScopeData6  DataLoggingSaveFormat=Array
  Vab_VSC : Scope
      settings: ActiveDisplayYMinimum=-833.7525  ActiveDisplayYMaximum=1202.9579  DataLoggingDecimation=10  DataLoggingVariableName=ScopeData7  DataLoggingSaveFormat=Array
  Vdc Boost : Display
      settings: Format=bank  Decimation=2000
  Vdc Inverter : Display
      settings: Format=bank  Decimation=2000
  W2kW : Gain  Gain=1/1000
  tag scope: Ia_B5=global, P_B1_kW_5=global, Va_B5=global
  wires:
  Selector/1 -> [Va_B5]
  [IdIq_prim_5] -> Demux/1
  [D_5] -> PV/5  "Duty Cycle"
  Pv/2(V) -> Vdc Boost/1, PV/4  "Vmean (V)"
  Selector1/1 -> [Ia_B5]
  [Temp_5] -> PV/2  "Temp (deg. C)"
  [Id_ref_5] -> Mux/1
  Power (Positive-Sequence)/2 -> Terminator1/1
  Pv/1(P) -> "P (kW) "/1, PV/3  "Pmean  (kW)"
  Power (Positive-Sequence)/1 -> W2kW/1
  [Va_B5] -> Grid/1  "Va (V)"
  [P_B1_kW_5] -> P_B1/1, P (kW)/1  "P (kW)"
  [Iabc_B5] -> Power (Positive-Sequence)/2, Selector1/1
  [Vab_VSC_5] -> Vab_VSC/1
  Demux/2 -> IdIq (pu) VSC Control/2  "Iq"
  Subsystem2/2(VrVm) -> VSC/1  "Vref - Vmean"
  [Vabc_B5] -> Power (Positive-Sequence)/1, Selector/1
  [m_5] -> VSC/2  "Mod. Index"
  Subsystem2/1(Vm) -> Vdc Inverter/1
  [V_PV_5] -> PV1/1  "V_PV"
  [I_PV_5] -> PV1/2  "I_PV"
  Mux/1 -> IdIq (pu) VSC Control/1  "Idref Id (magenta)"
  [Ia_B5] -> Grid/2  "Ia (A)"
  Demux/1 -> Mux/2
  W2kW/1 -> [P_B1_kW_5]
  [Ir_5] -> PV/1  "Ir (W/m^2)"
  [Idiode_PV_5] -> PV1/3  "Idiode_PV"

== system aIEEE13bus_with_solar_13bus_pl_1day/Subsystem645/VSC Control ==
  note: VSC Main Controller
  Vabc_prim : Inport  PortDimensions=3
  Iabc_prim : Inport  Port=2  PortDimensions=3
  Vdc_mes : Inport  Port=3  PortDimensions=1
  Current Regulator : Subsystem
  Iq_ref : Constant  Value=0
  Mux : Mux  Inputs=2
  PLL & Measurements : Subsystem
  PWM Generator (3-Level) : spsPWMGenerator3LevelLib/PWM Generator (3-Level)  ModulatorType=Three-phase bridge (12 pulses)  ModulatorMode=Unsynchronized  nF=27  Fc=33*60  ModulatingSignals=off  m=0.8  Freq=60  Phase=0  Ts=Ts_Power
  Uabc_ref Generation max (m) = 1 : Subsystem
  Unit Delay : UnitDelay  SampleTime=Ts_Control  HasFrameUpgradeWarning=on
  VDC Regulator : Subsystem
  Vdc_ref1 : Constant  Value=Vdc_ref
  Pulses : Outport  VectorParamsAs1DForOutWhenUnconnected=off
  wires:
  VDC Regulator/1(Id_ref) -> Mux/1
  PLL & Measurements/1(wt) -> Uabc_ref Generation max (m) = 1/1(wt)
  Current Regulator/1(VdVq_conv) -> Uabc_ref Generation max (m) = 1/2(VdVq_conv)
  Iq_ref/1 -> Mux/2
  Mux/1 -> Current Regulator/3(IdIq_ref)
  PLL & Measurements/3(IdIq_prim) -> Current Regulator/2(IdIq_mes)
  PLL & Measurements/2(VdVq_prim) -> Current Regulator/1(VdVq_mes)
  Vdc_mes/1 -> VDC Regulator/1(Vdc_mes)
  Vabc_prim/1 -> PLL & Measurements/1(Vabc_prim)
  Iabc_prim/1 -> PLL & Measurements/2(Iabc_prim)
  Unit Delay/1 -> PWM Generator (3-Level)/1
  PWM Generator (3-Level)/1 -> Pulses/1
  Uabc_ref Generation max (m) = 1/1(Uabc_ref) -> Unit Delay/1
  Vdc_ref1/1 -> VDC Regulator/2(Vdc_ref)

== system aIEEE13bus_with_solar_13bus_pl_1day/Subsystem646/B7 ==
  Kv : Gain  Gain=Ki  SaturateOnIntegerOverflow=on  OutDataTypeStr=Inherit: Same as input  ParamDataTypeStr=Inherit: Same as input
  Kv1 : Gain  Gain=Kv  SaturateOnIntegerOverflow=on  OutDataTypeStr=Inherit: Same as input  ParamDataTypeStr=Inherit: Same as input
  Mode I : spsVIMeasurementModel/Complex  SystemSampleTime=-1  VariantActivationTime=update diagram  EmptyChoice=off  PassThrough=off  PassThroughVariantControl=(default)  EmptyChoiceVariantControl=(default)  AllowFlexibleInterface=on  Latency=0  AutoFrameSizeCalculation=off
  Mode V : spsVIMeasurementModel/Complex  SystemSampleTime=-1  VariantActivationTime=update diagram  EmptyChoice=off  PassThrough=off  PassThroughVariantControl=(default)  EmptyChoiceVariantControl=(default)  AllowFlexibleInterface=on  Latency=0  AutoFrameSizeCalculation=off
  Model : spsVIMeasurementModel/VI  SystemSampleTime=-1  VariantActivationTime=update diagram  EmptyChoice=off  PassThrough=off  PassThroughVariantControl=(default)  EmptyChoiceVariantControl=(default)  AllowFlexibleInterface=on  Latency=0  AutoFrameSizeCalculation=off
  A : PMIOPort  Side=Left
  B : PMIOPort  Port=2  Side=Left
  C : PMIOPort  Port=3  Side=Left
  a : PMIOPort  Port=4  Side=Right
  b : PMIOPort  Port=5  Side=Right
  c : PMIOPort  Port=6  Side=Right
  tag scope: Iabc_B7=global, Vabc_B7=global
  wires:
  Mode V/1 -> [Vabc_B7]
  Mode I/1 -> [Iabc_B7]
  Kv1/1 -> Mode V/1
  Kv/1 -> Mode I/1
  Model/1 -> Kv1/1
  Model/2 -> Kv/1
  connections:
  Model/LConn2 -- B/RConn1
  Model/LConn1 -- A/RConn1
  Model/LConn3 -- C/RConn1
  Model/RConn2 -- b/RConn1
  Model/RConn1 -- a/RConn1
  Model/RConn3 -- c/RConn1

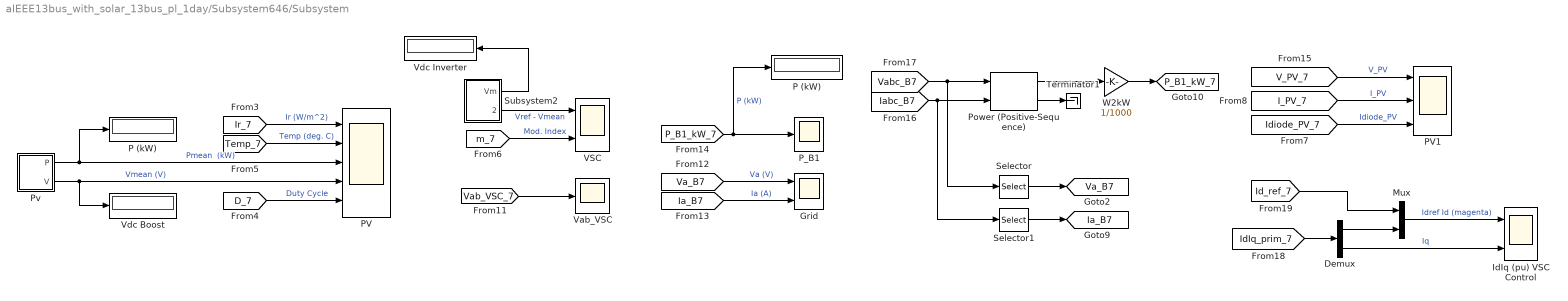
== system aIEEE13bus_with_solar_13bus_pl_1day/Subsystem646/Subsystem ==
  Demux : Demux  Outputs=2
  Grid : Scope  NumInputPorts=2
      settings: TimeSpan=0.05  ActiveDisplayYMinimum=-15250.872  ActiveDisplayYMaximum=15249.0697  DataLoggingDecimation=20  DataLoggingSaveFormat=Array
  IdIq (pu) VSC Control : Scope  NumInputPorts=2
      settings: TimeSpan=2  ActiveDisplayYMinimum=-5  ActiveDisplayYMaximum=5  DataLoggingDecimation=100  DataLoggingVariableName=ScopeData2  DataLoggingSaveFormat=Array
  Mux : Mux  Inputs=2
  P (kW) : Display
      settings: Format=bank  Decimation=2000
  "P (kW) " : Display
      settings: Format=bank  Decimation=2000
  PV : Scope  NumInputPorts=5
      settings: TimeSpan=2.5  ActiveDisplayYMinimum=156.25  ActiveDisplayYMaximum=1093.75  DataLoggingDecimation=100  DataLoggingVariableName=ScopeData3  DataLoggingSaveFormat=Array
  PV1 : Scope  NumInputPorts=3
      settings: TimeSpan=2  ActiveDisplayYMinimum=-37.8929  ActiveDisplayYMaximum=360.8644  DataLoggingDecimation=100  DataLoggingVariableName=ScopeData4  DataLoggingSaveFormat=Array
  P_B1 : Scope
      settings: TimeSpan=2.5  ActiveDisplayYMinimum=-54.8007  ActiveDisplayYMaximum=191.472  DataLoggingDecimation=100  DataLoggingVariableName=ScopeData5  DataLoggingSaveFormat=Array
  Power (Positive-Sequence) : spsPowerPositiveSequenceLib/Power (Positive-Sequence)  Freq=60  Vinit=[0, 0]  Iinit=[0, 0]  Ts=Ts_Control
  Pv : Subsystem
  Selector : Selector  InputPortWidth=3  IndexOptions=Index vector (dialog)  Indices=[1]  OutputSizes=1
  Selector1 : Selector  InputPortWidth=3  IndexOptions=Index vector (dialog)  Indices=[1]  OutputSizes=1
  Subsystem2 : Subsystem
  Terminator1 : Terminator
  VSC : Scope  NumInputPorts=2
      settings: TimeSpan=2.5  ActiveDisplayYMinimum=-145.1969  ActiveDisplayYMaximum=1306.7724  DataLoggingDecimation=100  DataLoggingVariableName=ScopeData6  DataLoggingSaveFormat=Array
  Vab_VSC : Scope
      settings: ActiveDisplayYMinimum=-833.7525  ActiveDisplayYMaximum=1202.9579  DataLoggingDecimation=10  DataLoggingVariableName=ScopeData7  DataLoggingSaveFormat=Array
  Vdc Boost : Display
      settings: Format=bank  Decimation=2000
  Vdc Inverter : Display
      settings: Format=bank  Decimation=2000
  W2kW : Gain  Gain=1/1000
  tag scope: Ia_B7=global, P_B1_kW_7=global, Va_B7=global
  wires:
  Selector/1 -> [Va_B7]
  [IdIq_prim_7] -> Demux/1
  [D_7] -> PV/5  "Duty Cycle"
  Pv/2(V) -> Vdc Boost/1, PV/4  "Vmean (V)"
  Selector1/1 -> [Ia_B7]
  [Temp_7] -> PV/2  "Temp (deg. C)"
  [Id_ref_7] -> Mux/1
  Power (Positive-Sequence)/2 -> Terminator1/1
  Pv/1(P) -> "P (kW) "/1, PV/3  "Pmean  (kW)"
  Power (Positive-Sequence)/1 -> W2kW/1
  [Va_B7] -> Grid/1  "Va (V)"
  [P_B1_kW_7] -> P_B1/1, P (kW)/1  "P (kW)"
  [Iabc_B7] -> Power (Positive-Sequence)/2, Selector1/1
  [Vab_VSC_7] -> Vab_VSC/1
  Demux/2 -> IdIq (pu) VSC Control/2  "Iq"
  Subsystem2/2(VrVm) -> VSC/1  "Vref - Vmean"
  [Vabc_B7] -> Power (Positive-Sequence)/1, Selector/1
  [m_7] -> VSC/2  "Mod. Index"
  Subsystem2/1(Vm) -> Vdc Inverter/1
  [V_PV_7] -> PV1/1  "V_PV"
  [I_PV_7] -> PV1/2  "I_PV"
  Mux/1 -> IdIq (pu) VSC Control/1  "Idref Id (magenta)"
  [Ia_B7] -> Grid/2  "Ia (A)"
  Demux/1 -> Mux/2
  W2kW/1 -> [P_B1_kW_7]
  [Ir_7] -> PV/1  "Ir (W/m^2)"
  [Idiode_PV_7] -> PV1/3  "Idiode_PV"

== system aIEEE13bus_with_solar_13bus_pl_1day/Subsystem646/VSC Control ==
  note: VSC Main Controller
  Vabc_prim : Inport  PortDimensions=3
  Iabc_prim : Inport  Port=2  PortDimensions=3
  Vdc_mes : Inport  Port=3  PortDimensions=1
  Current Regulator : Subsystem
  Iq_ref : Constant  Value=0
  Mux : Mux  Inputs=2
  PLL & Measurements : Subsystem
  PWM Generator (3-Level) : spsPWMGenerator3LevelLib/PWM Generator (3-Level)  ModulatorType=Three-phase bridge (12 pulses)  ModulatorMode=Unsynchronized  nF=27  Fc=33*60  ModulatingSignals=off  m=0.8  Freq=60  Phase=0  Ts=Ts_Power
  Uabc_ref Generation max (m) = 1 : Subsystem
  Unit Delay : UnitDelay  SampleTime=Ts_Control  HasFrameUpgradeWarning=on
  VDC Regulator : Subsystem
  Vdc_ref1 : Constant  Value=Vdc_ref
  Pulses : Outport  VectorParamsAs1DForOutWhenUnconnected=off
  wires:
  VDC Regulator/1(Id_ref) -> Mux/1
  PLL & Measurements/1(wt) -> Uabc_ref Generation max (m) = 1/1(wt)
  Current Regulator/1(VdVq_conv) -> Uabc_ref Generation max (m) = 1/2(VdVq_conv)
  Iq_ref/1 -> Mux/2
  Mux/1 -> Current Regulator/3(IdIq_ref)
  PLL & Measurements/3(IdIq_prim) -> Current Regulator/2(IdIq_mes)
  PLL & Measurements/2(VdVq_prim) -> Current Regulator/1(VdVq_mes)
  Vdc_mes/1 -> VDC Regulator/1(Vdc_mes)
  Vabc_prim/1 -> PLL & Measurements/1(Vabc_prim)
  Iabc_prim/1 -> PLL & Measurements/2(Iabc_prim)
  Unit Delay/1 -> PWM Generator (3-Level)/1
  PWM Generator (3-Level)/1 -> Pulses/1
  Uabc_ref Generation max (m) = 1/1(Uabc_ref) -> Unit Delay/1
  Vdc_ref1/1 -> VDC Regulator/2(Vdc_ref)

== system aIEEE13bus_with_solar_13bus_pl_1day/Subsystem652/B6 ==
  Kv : Gain  Gain=Ki  SaturateOnIntegerOverflow=on  OutDataTypeStr=Inherit: Same as input  ParamDataTypeStr=Inherit: Same as input
  Kv1 : Gain  Gain=Kv  SaturateOnIntegerOverflow=on  OutDataTypeStr=Inherit: Same as input  ParamDataTypeStr=Inherit: Same as input
  Mode I : spsVIMeasurementModel/Complex  SystemSampleTime=-1  VariantActivationTime=update diagram  EmptyChoice=off  PassThrough=off  PassThroughVariantControl=(default)  EmptyChoiceVariantControl=(default)  AllowFlexibleInterface=on  Latency=0  AutoFrameSizeCalculation=off
  Mode V : spsVIMeasurementModel/Complex  SystemSampleTime=-1  VariantActivationTime=update diagram  EmptyChoice=off  PassThrough=off  PassThroughVariantControl=(default)  EmptyChoiceVariantControl=(default)  AllowFlexibleInterface=on  Latency=0  AutoFrameSizeCalculation=off
  Model : spsVIMeasurementModel/VI  SystemSampleTime=-1  VariantActivationTime=update diagram  EmptyChoice=off  PassThrough=off  PassThroughVariantControl=(default)  EmptyChoiceVariantControl=(default)  AllowFlexibleInterface=on  Latency=0  AutoFrameSizeCalculation=off
  A : PMIOPort  Side=Left
  B : PMIOPort  Port=2  Side=Left
  C : PMIOPort  Port=3  Side=Left
  a : PMIOPort  Port=4  Side=Right
  b : PMIOPort  Port=5  Side=Right
  c : PMIOPort  Port=6  Side=Right
  tag scope: Iabc_B6=global, Vabc_B6=global
  wires:
  Mode V/1 -> [Vabc_B6]
  Mode I/1 -> [Iabc_B6]
  Kv1/1 -> Mode V/1
  Kv/1 -> Mode I/1
  Model/1 -> Kv1/1
  Model/2 -> Kv/1
  connections:
  Model/LConn2 -- B/RConn1
  Model/LConn1 -- A/RConn1
  Model/LConn3 -- C/RConn1
  Model/RConn2 -- b/RConn1
  Model/RConn1 -- a/RConn1
  Model/RConn3 -- c/RConn1

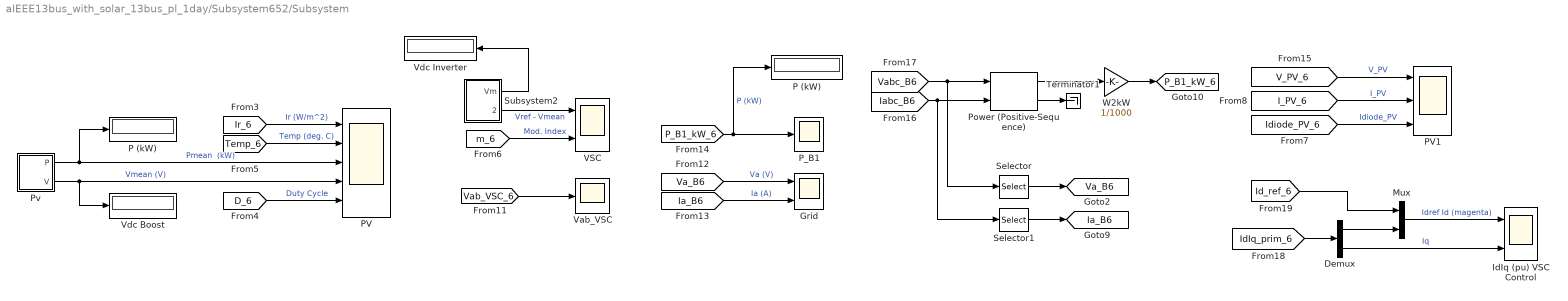
== system aIEEE13bus_with_solar_13bus_pl_1day/Subsystem652/Subsystem ==
  Demux : Demux  Outputs=2
  Grid : Scope  NumInputPorts=2
      settings: TimeSpan=0.05  ActiveDisplayYMinimum=-15250.872  ActiveDisplayYMaximum=15249.0697  DataLoggingDecimation=20  DataLoggingSaveFormat=Array
  IdIq (pu) VSC Control : Scope  NumInputPorts=2
      settings: TimeSpan=2  ActiveDisplayYMinimum=-5  ActiveDisplayYMaximum=5  DataLoggingDecimation=100  DataLoggingVariableName=ScopeData2  DataLoggingSaveFormat=Array
  Mux : Mux  Inputs=2
  P (kW) : Display
      settings: Format=bank  Decimation=2000
  "P (kW) " : Display
      settings: Format=bank  Decimation=2000
  PV : Scope  NumInputPorts=5
      settings: TimeSpan=2.5  ActiveDisplayYMinimum=156.25  ActiveDisplayYMaximum=1093.75  DataLoggingDecimation=100  DataLoggingVariableName=ScopeData3  DataLoggingSaveFormat=Array
  PV1 : Scope  NumInputPorts=3
      settings: TimeSpan=2  ActiveDisplayYMinimum=-37.8929  ActiveDisplayYMaximum=360.8644  DataLoggingDecimation=100  DataLoggingVariableName=ScopeData4  DataLoggingSaveFormat=Array
  P_B1 : Scope
      settings: TimeSpan=2.5  ActiveDisplayYMinimum=-54.8007  ActiveDisplayYMaximum=191.472  DataLoggingDecimation=100  DataLoggingVariableName=ScopeData5  DataLoggingSaveFormat=Array
  Power (Positive-Sequence) : spsPowerPositiveSequenceLib/Power (Positive-Sequence)  Freq=60  Vinit=[0, 0]  Iinit=[0, 0]  Ts=Ts_Control
  Pv : Subsystem
  Selector : Selector  InputPortWidth=3  IndexOptions=Index vector (dialog)  Indices=[1]  OutputSizes=1
  Selector1 : Selector  InputPortWidth=3  IndexOptions=Index vector (dialog)  Indices=[1]  OutputSizes=1
  Subsystem2 : Subsystem
  Terminator1 : Terminator
  VSC : Scope  NumInputPorts=2
      settings: TimeSpan=2.5  ActiveDisplayYMinimum=-145.1969  ActiveDisplayYMaximum=1306.7724  DataLoggingDecimation=100  DataLoggingVariableName=ScopeData6  DataLoggingSaveFormat=Array
  Vab_VSC : Scope
      settings: ActiveDisplayYMinimum=-833.7525  ActiveDisplayYMaximum=1202.9579  DataLoggingDecimation=10  DataLoggingVariableName=ScopeData7  DataLoggingSaveFormat=Array
  Vdc Boost : Display
      settings: Format=bank  Decimation=2000
  Vdc Inverter : Display
      settings: Format=bank  Decimation=2000
  W2kW : Gain  Gain=1/1000
  tag scope: Ia_B6=global, P_B1_kW_6=global, Va_B6=global
  wires:
  Selector/1 -> [Va_B6]
  [IdIq_prim_6] -> Demux/1
  [D_6] -> PV/5  "Duty Cycle"
  Pv/2(V) -> Vdc Boost/1, PV/4  "Vmean (V)"
  Selector1/1 -> [Ia_B6]
  [Temp_6] -> PV/2  "Temp (deg. C)"
  [Id_ref_6] -> Mux/1
  Power (Positive-Sequence)/2 -> Terminator1/1
  Pv/1(P) -> "P (kW) "/1, PV/3  "Pmean  (kW)"
  Power (Positive-Sequence)/1 -> W2kW/1
  [Va_B6] -> Grid/1  "Va (V)"
  [P_B1_kW_6] -> P_B1/1, P (kW)/1  "P (kW)"
  [Iabc_B6] -> Power (Positive-Sequence)/2, Selector1/1
  [Vab_VSC_6] -> Vab_VSC/1
  Demux/2 -> IdIq (pu) VSC Control/2  "Iq"
  Subsystem2/2(VrVm) -> VSC/1  "Vref - Vmean"
  [Vabc_B6] -> Power (Positive-Sequence)/1, Selector/1
  [m_6] -> VSC/2  "Mod. Index"
  Subsystem2/1(Vm) -> Vdc Inverter/1
  [V_PV_6] -> PV1/1  "V_PV"
  [I_PV_6] -> PV1/2  "I_PV"
  Mux/1 -> IdIq (pu) VSC Control/1  "Idref Id (magenta)"
  [Ia_B6] -> Grid/2  "Ia (A)"
  Demux/1 -> Mux/2
  W2kW/1 -> [P_B1_kW_6]
  [Ir_6] -> PV/1  "Ir (W/m^2)"
  [Idiode_PV_6] -> PV1/3  "Idiode_PV"

== system aIEEE13bus_with_solar_13bus_pl_1day/Subsystem652/VSC Control ==
  note: VSC Main Controller
  Vabc_prim : Inport  PortDimensions=3
  Iabc_prim : Inport  Port=2  PortDimensions=3
  Vdc_mes : Inport  Port=3  PortDimensions=1
  Current Regulator : Subsystem
  Iq_ref : Constant  Value=0
  Mux : Mux  Inputs=2
  PLL & Measurements : Subsystem
  PWM Generator (3-Level) : spsPWMGenerator3LevelLib/PWM Generator (3-Level)  ModulatorType=Three-phase bridge (12 pulses)  ModulatorMode=Unsynchronized  nF=27  Fc=33*60  ModulatingSignals=off  m=0.8  Freq=60  Phase=0  Ts=Ts_Power
  Uabc_ref Generation max (m) = 1 : Subsystem
  Unit Delay : UnitDelay  SampleTime=Ts_Control  HasFrameUpgradeWarning=on
  VDC Regulator : Subsystem
  Vdc_ref1 : Constant  Value=Vdc_ref
  Pulses : Outport  VectorParamsAs1DForOutWhenUnconnected=off
  wires:
  VDC Regulator/1(Id_ref) -> Mux/1
  PLL & Measurements/1(wt) -> Uabc_ref Generation max (m) = 1/1(wt)
  Current Regulator/1(VdVq_conv) -> Uabc_ref Generation max (m) = 1/2(VdVq_conv)
  Iq_ref/1 -> Mux/2
  Mux/1 -> Current Regulator/3(IdIq_ref)
  PLL & Measurements/3(IdIq_prim) -> Current Regulator/2(IdIq_mes)
  PLL & Measurements/2(VdVq_prim) -> Current Regulator/1(VdVq_mes)
  Vdc_mes/1 -> VDC Regulator/1(Vdc_mes)
  Vabc_prim/1 -> PLL & Measurements/1(Vabc_prim)
  Iabc_prim/1 -> PLL & Measurements/2(Iabc_prim)
  Unit Delay/1 -> PWM Generator (3-Level)/1
  PWM Generator (3-Level)/1 -> Pulses/1
  Uabc_ref Generation max (m) = 1/1(Uabc_ref) -> Unit Delay/1
  Vdc_ref1/1 -> VDC Regulator/2(Vdc_ref)
